simulink model "s5_Inverter_PSMG"  (R2019b)
settings: Solver=VariableStepAuto  StartTime=0.0  StopTime=10.0  RelTol=1e-3
libraries: powerlib x41, powerlib_meascontrol x7, simulink_extras x1
settings Model: Creator=MAHMUD  LastModifiedBy=MAHMUD

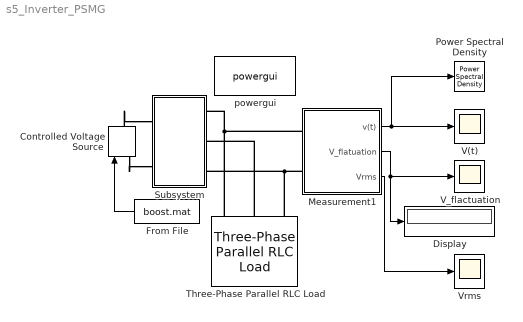
== system s5_Inverter_PSMG ==
  Controlled Voltage Source : powerlib/Electrical Sources/Controlled Voltage Source  Initialize=on  Source_Type=DC  Amplitude=0  Phase=0  Frequency=0  Measurements=None
      settings: SourceProductName=Simscape Electrical
  Display : Display
  From File : FromFile  FileName=boost.mat
  Measurement1 : Subsystem
  Power Spectral Density : simulink_extras/Additional Sinks/Power Spectral Density  npts=5000  fftpts=512  HowOften=500  sampleT=0.001
      settings: SourceProductName=Simulink  SourceProductBaseCode=SL
  Subsystem : Subsystem
  Three-Phase Parallel RLC Load : powerlib/Elements/Three-Phase Parallel RLC Load  LConnTagsString=A|B|C  Configuration=Y (grounded)  NominalVoltage=1000  Vabc=[1e3 1e3 1e3]  Vabcp=[1e3 1e3 1e3]  NominalFrequency=50  UnbalancedPower=off  ActivePower=16e3  InductivePower=100  CapacitivePower=100  Pabc=[10e3 9e3 11e3]  QLabc=[100 90 110]  QCabc=[100 90 110]  Pabcp=[10e3 9e3 11e3]  QLabcp=[100 90 110]  QCabcp=[100 90 110]  Measurements=None  LoadType=constant Z
      settings: SourceProductName=Simscape Electrical
  V(t) : Scope
  V_flactuation : Scope
  Vrms : Scope
  powergui : powerlib/powergui  Priority=1  SimulationMode=Continuous  SampleTime=50e-6  frequency=60  Iterations=50  frequencyindice=0  Pbase=100e6  ErrMax=1e-4  UnitsV=kV  UnitsW=MW  buscounter=0  FunctionMessages=off  echomessages=off  EnableUseOfTLC=off  CurrentSourceSwitches=off  DisableSnubberDevices=off  DisableRonSwitches=off  DisableVfSwitches=off  DisplayEquations=off  AutomaticDiscreteSolvers=off  SolverType=Tustin/Backward Euler (TBE)  Interpol=off  ExternalGateDelay=off  methode=off  Ts=100  x0status=blocks  SPID=on  SwTol=0  HookPort=off  NonlinearTolerance=1e-4  nMaxIteration=100  ContinueOnMaxIteration=off  RestoreLinks=warning  ResistiveCurrentMeasurement=off  Frange=[0:2:500]  Ylog=off  Xlog=on  ShowGrid=off  save=off  variable=ZData  structure=0  ZoomFFT=off  StartTime=0.0  cycles=1  DisplayStyle=1  fundamental=60  FreqAxis=off  MaxFrequency=1000  frequencyindicesteady=1  RmsSteady=1  display=off
      settings: SourceProductName=Simscape Electrical
  wires:
  From File/1 -> Controlled Voltage Source/1
  Measurement1/3(Vrms) -> Vrms/1
  Measurement1/2(V_flatuation) -> Display/1, V_flactuation/1
  Measurement1/1(v(t)) -> V(t)/1, Power Spectral Density/1
  connections:
  Controlled Voltage Source/RConn1 -- Subsystem/LConn1
  Controlled Voltage Source/LConn1 -- Subsystem/LConn2
  Three-Phase Parallel RLC Load/LConn1 -- Subsystem/RConn1 -- Measurement1/LConn1
  Three-Phase Parallel RLC Load/LConn2 -- Subsystem/RConn2
  Three-Phase Parallel RLC Load/LConn3 -- Subsystem/RConn3 -- Measurement1/LConn2

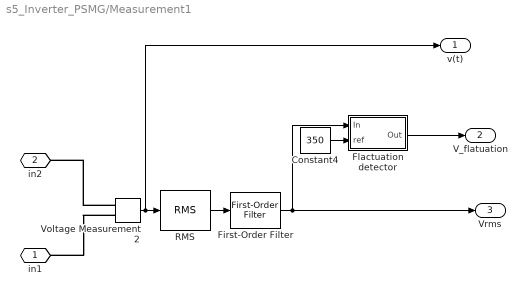
== system s5_Inverter_PSMG/Measurement1 ==
  Constant4 : Constant  Value=350
  First-Order Filter : powerlib_meascontrol/Filters/First-Order Filter  FilterType=Lowpass  Tc=100e-3  Ts=0  Initialize=off  Vac_Init=[0, 0, 50]  Vdc_Init=0  PlotResponse=off  FreqRange="[0,  200,  1]"
      settings: SourceProductName=Simscape Electrical
  Flactuation detector : Subsystem
  RMS : powerlib_meascontrol/Measurements/RMS  TrueRMS=on  Freq=50  RMSInit=210  Ts=0.001
      settings: SourceProductName=Simscape Electrical
  Voltage Measurement2 : powerlib/Measurements/Voltage Measurement  PhasorSimulation=off  OutputType=Complex  PSBequivalent=0
      settings: SourceProductName=Simscape Electrical
  in1 : PMIOPort  Side=Left
  in2 : PMIOPort  Port=2  Side=Left
  v(t) : Outport
  V_flatuation : Outport  Port=2
  Vrms : Outport  Port=3
  wires:
  Voltage Measurement2/1 -> v(t)/1, RMS/1
  First-Order Filter/1 -> Vrms/1, Flactuation detector/1(In)
  RMS/1 -> First-Order Filter/1
  Flactuation detector/1(Out) -> V_flatuation/1
  Constant4/1 -> Flactuation detector/2(ref)
  connections:
  Voltage Measurement2/LConn2 -- in1/RConn1
  Voltage Measurement2/LConn1 -- in2/RConn1

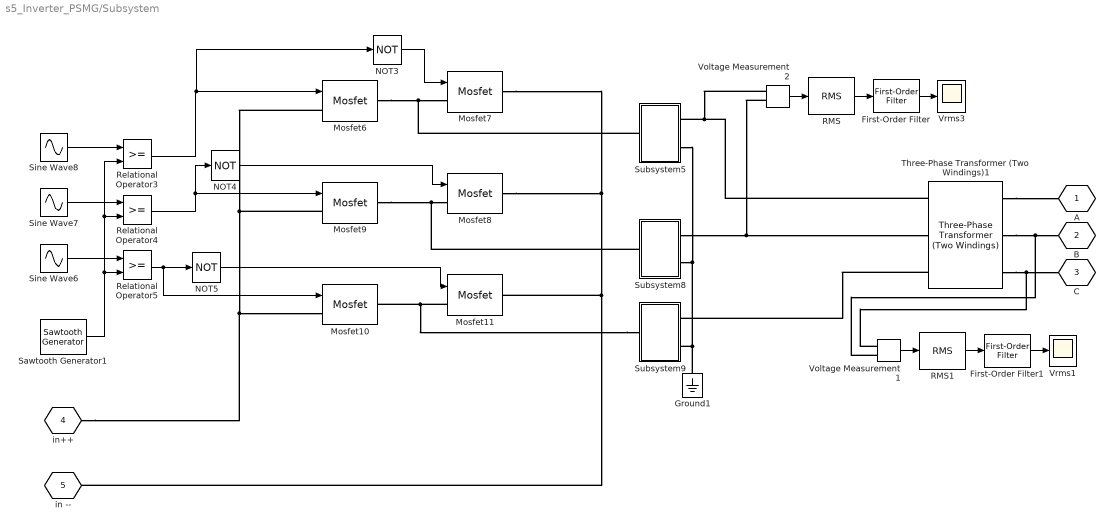
== system s5_Inverter_PSMG/Subsystem ==
  First-Order Filter : powerlib_meascontrol/Filters/First-Order Filter  FilterType=Lowpass  Tc=100e-3  Ts=0  Initialize=off  Vac_Init=[0, 0, 50]  Vdc_Init=0  PlotResponse=off  FreqRange="[0,  200,  1]"
      settings: SourceProductName=Simscape Electrical
  First-Order Filter1 : powerlib_meascontrol/Filters/First-Order Filter  FilterType=Lowpass  Tc=100e-3  Ts=0  Initialize=off  Vac_Init=[0, 0, 50]  Vdc_Init=0  PlotResponse=off  FreqRange="[0,  200,  1]"
      settings: SourceProductName=Simscape Electrical
  Ground1 : powerlib/Elements/Ground  LConnTagsString=a
      settings: SourceProductName=Simscape Electrical
  Mosfet{6..11} (6 alike) : powerlib/Power Electronics/Mosfet  Ron=0.1  Lon=0  Rd=0.01  Vfd=0  IC=0  Rs=1e5  Cs=inf  Measurements=off
      settings: SourceProductName=Simscape Electrical
  NOT3 : Logic  Operator=NOT  IconShape=distinctive  AllPortsSameDT=off  OutDataTypeStr=boolean
  NOT4 : Logic  Operator=NOT  IconShape=distinctive  AllPortsSameDT=off  OutDataTypeStr=boolean
  NOT5 : Logic  Operator=NOT  IconShape=distinctive  AllPortsSameDT=off  OutDataTypeStr=boolean
  RMS : powerlib_meascontrol/Measurements/RMS  TrueRMS=on  Freq=50  RMSInit=210  Ts=0.001
      settings: SourceProductName=Simscape Electrical
  RMS1 : powerlib_meascontrol/Measurements/RMS  TrueRMS=on  Freq=50  RMSInit=210  Ts=0.001
      settings: SourceProductName=Simscape Electrical
  Relational Operator3 : RelationalOperator  OutDataTypeStr=boolean  ZeroCross=off  RndMeth=Simplest
  Relational Operator4 : RelationalOperator  OutDataTypeStr=boolean  ZeroCross=off  RndMeth=Simplest
  Relational Operator5 : RelationalOperator  OutDataTypeStr=boolean  ZeroCross=off  RndMeth=Simplest
  Sawtooth Generator1 : powerlib_meascontrol/Pulse & Signal Generators/Sawtooth Generator  Freq=1e3  Phase=180  Ts=0
      settings: SourceProductName=Simscape Electrical
  Sine Wave6 : Sin  Frequency=2*pi*50  Phase=4*pi/3  SampleTime=0
  Sine Wave7 : Sin  Frequency=2*pi*50  Phase=2*pi/3  SampleTime=0
  Sine Wave8 : Sin  Frequency=2*pi*50  SampleTime=0
  Subsystem5 : Subsystem
  Subsystem8 : Subsystem
  Subsystem9 : Subsystem
  Three-Phase Transformer (Two Windings)1 : powerlib/Elements/Three-Phase Transformer (Two Windings)  Winding1Connection=Yg  Winding2Connection=Yg  CoreType=Three single-phase transformers  SetSaturation=off  Hysteresis=off  DataFile='hysteresis'  SetInitialFlux=off  Measurements=None  UNITS=pu  NominalPower=[ 16e3 , 50 ]  Winding1=[ 80 , 0.002 , 0.08 ]  Winding2=[ 400 , 0.002 , 0.08 ]  Rm=500  Lm=500  L0=0.5  Saturation=[ 0,0 ; 0.0024,1.2 ; 1.0,1.52 ]  InitialFluxes=[ 0.8 , -0.8 , 0.7 ]  BreakLoop=off  DiscreteSolver=Trapezoidal iterative  DataType=off  TransfoNumber=1
      settings: SourceProductName=Simscape Electrical
  Voltage Measurement1 : powerlib/Measurements/Voltage Measurement  PhasorSimulation=off  OutputType=Complex  PSBequivalent=0
      settings: SourceProductName=Simscape Electrical
  Voltage Measurement2 : powerlib/Measurements/Voltage Measurement  PhasorSimulation=off  OutputType=Complex  PSBequivalent=0
      settings: SourceProductName=Simscape Electrical
  Vrms1 : Scope
  Vrms3 : Scope
  A : PMIOPort  Tag=PMCPort  Side=Right
  B : PMIOPort  Tag=PMCPort  Port=2  Side=Right
  C : PMIOPort  Tag=PMCPort  Port=3  Side=Right
  in++ : PMIOPort  Tag=PMCPort  Port=4  Side=Left
  in -- : PMIOPort  Tag=PMCPort  Port=5  Side=Left
  wires:
  Relational Operator3/1 -> NOT3/1, Mosfet6/1
  Sine Wave7/1 -> Relational Operator4/1
  NOT4/1 -> Mosfet8/1
  Relational Operator5/1 -> Mosfet10/1, NOT5/1
  Relational Operator4/1 -> Mosfet9/1, NOT4/1
  Sine Wave8/1 -> Relational Operator3/1
  NOT5/1 -> Mosfet11/1
  NOT3/1 -> Mosfet7/1
  Sine Wave6/1 -> Relational Operator5/1
  Sawtooth Generator1/1 -> Relational Operator3/2, Relational Operator4/2, Relational Operator5/2
  Voltage Measurement2/1 -> RMS/1
  RMS/1 -> First-Order Filter/1
  First-Order Filter/1 -> Vrms3/1
  First-Order Filter1/1 -> Vrms1/1
  RMS1/1 -> First-Order Filter1/1
  Voltage Measurement1/1 -> RMS1/1
  connections:
  Subsystem5/RConn2 -- Ground1/LConn1 -- Subsystem9/RConn2 -- Subsystem8/RConn2
  Three-Phase Transformer (Two Windings)1/LConn3 -- Subsystem9/RConn1
  Subsystem8/LConn1 -- Mosfet9/RConn1 -- Mosfet8/LConn1
  Subsystem5/LConn1 -- Mosfet6/RConn1 -- Mosfet7/LConn1
  Mosfet6/LConn1 -- in++/RConn1 -- Mosfet10/LConn1 -- Mosfet9/LConn1
  Subsystem9/LConn1 -- Mosfet11/LConn1 -- Mosfet10/RConn1
  Mosfet11/RConn1 -- in --/RConn1 -- Mosfet7/RConn1 -- Mosfet8/RConn1
  Three-Phase Transformer (Two Windings)1/RConn2 -- Voltage Measurement1/LConn2 -- B/RConn1
  Three-Phase Transformer (Two Windings)1/LConn1 -- Voltage Measurement2/LConn1 -- Subsystem5/RConn1
  Subsystem8/RConn1 -- Voltage Measurement2/LConn2 -- Three-Phase Transformer (Two Windings)1/LConn2
  Three-Phase Transformer (Two Windings)1/RConn3 -- Voltage Measurement1/LConn1 -- C/RConn1
  Three-Phase Transformer (Two Windings)1/RConn1 -- A/RConn1

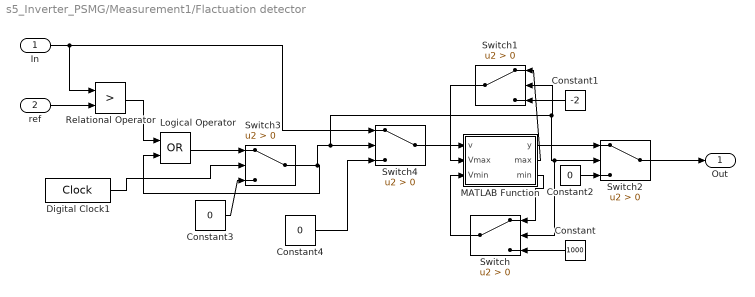
== system s5_Inverter_PSMG/Measurement1/Flactuation detector ==
  In : Inport
  ref : Inport  Port=2
  Constant : Constant  Value=1000
  Constant1 : Constant  Value=-2
  Constant2 : Constant  Value=0
  Constant3 : Constant  Value=0
  Constant4 : Constant  Value=0
  Digital Clock1 : DigitalClock
  Logical Operator : Logic  Operator=OR  AllPortsSameDT=off  OutDataTypeStr=boolean
  MATLAB Function : MATLAB Function  TreatAsAtomicUnit=on
  Relational Operator : RelationalOperator  Operator=>  OutDataTypeStr=boolean  ZeroCross=off  RndMeth=Simplest
  Switch{,1..4} (5 alike) : Switch  Criteria=u2 > Threshold  ZeroCross=off
  Out : Outport
  wires:
  Constant/1 -> Switch/3
  Switch1/1 -> MATLAB Function/2(Vmax)
  Constant1/1 -> Switch1/3
  MATLAB Function/1(y) -> Switch2/1
  MATLAB Function/3(min) -> Switch/1
  Switch2/1 -> Out/1
  MATLAB Function/2(max) -> Switch1/1
  Switch/1 -> MATLAB Function/3(Vmin)
  Constant2/1 -> Switch2/3
  Logical Operator/1 -> Switch3/1
  Switch3/1 -> Switch/2, Switch2/2, Switch1/2, Switch4/2, Logical Operator/2
  Constant3/1 -> Switch3/3
  Relational Operator/1 -> Logical Operator/1
  Switch4/1 -> MATLAB Function/1(v)
  In/1 -> Relational Operator/1, Switch4/1
  Digital Clock1/1 -> Switch3/2
  ref/1 -> Relational Operator/2
  Constant4/1 -> Switch4/3

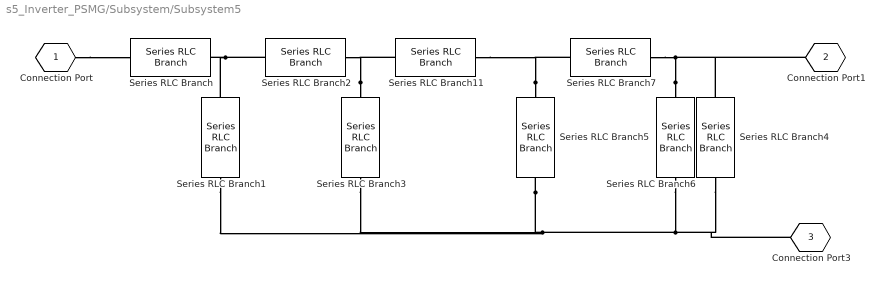
== system s5_Inverter_PSMG/Subsystem/Subsystem5 ==
  Series RLC Branch{,2,5..6} (4 alike) : powerlib/Elements/Series RLC Branch  LConnTagsString=__new0  RConnTagsString=__new0  BranchType=L  Resistance=1  Inductance=92e-3  SetiL0=off  InitialCurrent=0  Capacitance=1e-6  Setx0=off  InitialVoltage=0  Measurements=None
      settings: SourceProductName=Simscape Electrical
  Series RLC Branch1 : powerlib/Elements/Series RLC Branch  LConnTagsString=__new0  RConnTagsString=__new0  BranchType=C  Resistance=1  Inductance=1e-3  SetiL0=off  InitialCurrent=0  Capacitance=110e-6  Setx0=off  InitialVoltage=0  Measurements=None
      settings: SourceProductName=Simscape Electrical
  Series RLC Branch11 : powerlib/Elements/Series RLC Branch  LConnTagsString=__new0  RConnTagsString=__new0  BranchType=R  Resistance=1  Inductance=1e-3  SetiL0=off  InitialCurrent=0  Capacitance=110e-6  Setx0=off  InitialVoltage=0  Measurements=None
      settings: SourceProductName=Simscape Electrical
  Series RLC Branch3 : powerlib/Elements/Series RLC Branch  LConnTagsString=__new0  RConnTagsString=__new0  BranchType=R  Resistance=500  Inductance=1e-3  SetiL0=off  InitialCurrent=0  Capacitance=110e-6  Setx0=off  InitialVoltage=0  Measurements=None
      settings: SourceProductName=Simscape Electrical
  Series RLC Branch4 : powerlib/Elements/Series RLC Branch  LConnTagsString=__new0  RConnTagsString=__new0  BranchType=R  Resistance=10  Inductance=1e-3  SetiL0=off  InitialCurrent=0  Capacitance=110e-6  Setx0=off  InitialVoltage=0  Measurements=None
      settings: SourceProductName=Simscape Electrical
  Series RLC Branch7 : powerlib/Elements/Series RLC Branch  LConnTagsString=__new0  RConnTagsString=__new0  BranchType=C  Resistance=1  Inductance=1e-3  SetiL0=off  InitialCurrent=0  Capacitance=110e-6  Setx0=off  InitialVoltage=0  Measurements=None
      settings: SourceProductName=Simscape Electrical
  Connection Port : PMIOPort  Tag=PMCPort  Side=Left
  Connection Port1 : PMIOPort  Tag=PMCPort  Port=2  Side=Right
  Connection Port3 : PMIOPort  Tag=PMCPort  Port=3  Side=Right
  connections:
  Connection Port/RConn1 -- Series RLC Branch/LConn1
  Series RLC Branch/RConn1 -- Series RLC Branch2/LConn1 -- Series RLC Branch1/RConn1
  Series RLC Branch5/LConn1 -- Series RLC Branch11/RConn1 -- Series RLC Branch7/LConn1
  Series RLC Branch5/RConn1 -- Series RLC Branch6/RConn1 -- Series RLC Branch4/LConn1 -- Connection Port3/RConn1 -- Series RLC Branch3/LConn1 -- Series RLC Branch1/LConn1
  Series RLC Branch3/RConn1 -- Series RLC Branch11/LConn1 -- Series RLC Branch2/RConn1
  Series RLC Branch6/LConn1 -- Series RLC Branch4/RConn1 -- Connection Port1/RConn1 -- Series RLC Branch7/RConn1

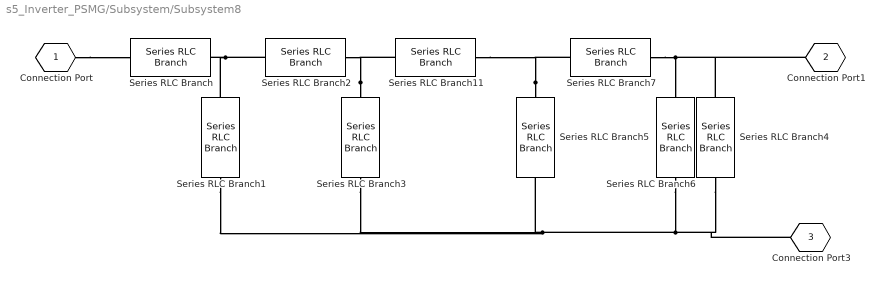
== system s5_Inverter_PSMG/Subsystem/Subsystem8 ==
  Series RLC Branch{,2,5..6} (4 alike) : powerlib/Elements/Series RLC Branch  LConnTagsString=__new0  RConnTagsString=__new0  BranchType=L  Resistance=1  Inductance=92e-3  SetiL0=off  InitialCurrent=0  Capacitance=1e-6  Setx0=off  InitialVoltage=0  Measurements=None
      settings: SourceProductName=Simscape Electrical
  Series RLC Branch1 : powerlib/Elements/Series RLC Branch  LConnTagsString=__new0  RConnTagsString=__new0  BranchType=C  Resistance=1  Inductance=1e-3  SetiL0=off  InitialCurrent=0  Capacitance=110e-6  Setx0=off  InitialVoltage=0  Measurements=None
      settings: SourceProductName=Simscape Electrical
  Series RLC Branch11 : powerlib/Elements/Series RLC Branch  LConnTagsString=__new0  RConnTagsString=__new0  BranchType=R  Resistance=1  Inductance=1e-3  SetiL0=off  InitialCurrent=0  Capacitance=110e-6  Setx0=off  InitialVoltage=0  Measurements=None
      settings: SourceProductName=Simscape Electrical
  Series RLC Branch3 : powerlib/Elements/Series RLC Branch  LConnTagsString=__new0  RConnTagsString=__new0  BranchType=R  Resistance=500  Inductance=1e-3  SetiL0=off  InitialCurrent=0  Capacitance=110e-6  Setx0=off  InitialVoltage=0  Measurements=None
      settings: SourceProductName=Simscape Electrical
  Series RLC Branch4 : powerlib/Elements/Series RLC Branch  LConnTagsString=__new0  RConnTagsString=__new0  BranchType=R  Resistance=10  Inductance=1e-3  SetiL0=off  InitialCurrent=0  Capacitance=110e-6  Setx0=off  InitialVoltage=0  Measurements=None
      settings: SourceProductName=Simscape Electrical
  Series RLC Branch7 : powerlib/Elements/Series RLC Branch  LConnTagsString=__new0  RConnTagsString=__new0  BranchType=C  Resistance=1  Inductance=1e-3  SetiL0=off  InitialCurrent=0  Capacitance=110e-6  Setx0=off  InitialVoltage=0  Measurements=None
      settings: SourceProductName=Simscape Electrical
  Connection Port : PMIOPort  Tag=PMCPort  Side=Left
  Connection Port1 : PMIOPort  Tag=PMCPort  Port=2  Side=Right
  Connection Port3 : PMIOPort  Tag=PMCPort  Port=3  Side=Right
  connections:
  Series RLC Branch7/RConn1 -- Series RLC Branch6/LConn1 -- Series RLC Branch4/RConn1 -- Connection Port1/RConn1
  Series RLC Branch3/RConn1 -- Series RLC Branch2/RConn1 -- Series RLC Branch11/LConn1
  Series RLC Branch6/RConn1 -- Series RLC Branch3/LConn1 -- Series RLC Branch1/LConn1 -- Series RLC Branch5/RConn1 -- Series RLC Branch4/LConn1 -- Connection Port3/RConn1
  Series RLC Branch5/LConn1 -- Series RLC Branch7/LConn1 -- Series RLC Branch11/RConn1
  Series RLC Branch1/RConn1 -- Series RLC Branch2/LConn1 -- Series RLC Branch/RConn1
  Connection Port/RConn1 -- Series RLC Branch/LConn1

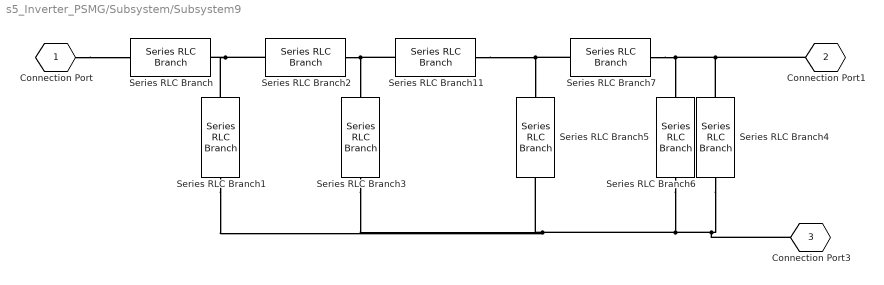
== system s5_Inverter_PSMG/Subsystem/Subsystem9 ==
  Series RLC Branch{,2,5..6} (4 alike) : powerlib/Elements/Series RLC Branch  LConnTagsString=__new0  RConnTagsString=__new0  BranchType=L  Resistance=1  Inductance=92e-3  SetiL0=off  InitialCurrent=0  Capacitance=1e-6  Setx0=off  InitialVoltage=0  Measurements=None
      settings: SourceProductName=Simscape Electrical
  Series RLC Branch1 : powerlib/Elements/Series RLC Branch  LConnTagsString=__new0  RConnTagsString=__new0  BranchType=C  Resistance=1  Inductance=1e-3  SetiL0=off  InitialCurrent=0  Capacitance=110e-6  Setx0=off  InitialVoltage=0  Measurements=None
      settings: SourceProductName=Simscape Electrical
  Series RLC Branch11 : powerlib/Elements/Series RLC Branch  LConnTagsString=__new0  RConnTagsString=__new0  BranchType=R  Resistance=1  Inductance=1e-3  SetiL0=off  InitialCurrent=0  Capacitance=110e-6  Setx0=off  InitialVoltage=0  Measurements=None
      settings: SourceProductName=Simscape Electrical
  Series RLC Branch3 : powerlib/Elements/Series RLC Branch  LConnTagsString=__new0  RConnTagsString=__new0  BranchType=R  Resistance=500  Inductance=1e-3  SetiL0=off  InitialCurrent=0  Capacitance=110e-6  Setx0=off  InitialVoltage=0  Measurements=None
      settings: SourceProductName=Simscape Electrical
  Series RLC Branch4 : powerlib/Elements/Series RLC Branch  LConnTagsString=__new0  RConnTagsString=__new0  BranchType=R  Resistance=10  Inductance=1e-3  SetiL0=off  InitialCurrent=0  Capacitance=110e-6  Setx0=off  InitialVoltage=0  Measurements=None
      settings: SourceProductName=Simscape Electrical
  Series RLC Branch7 : powerlib/Elements/Series RLC Branch  LConnTagsString=__new0  RConnTagsString=__new0  BranchType=C  Resistance=1  Inductance=1e-3  SetiL0=off  InitialCurrent=0  Capacitance=110e-6  Setx0=off  InitialVoltage=0  Measurements=None
      settings: SourceProductName=Simscape Electrical
  Connection Port : PMIOPort  Tag=PMCPort  Side=Left
  Connection Port1 : PMIOPort  Tag=PMCPort  Port=2  Side=Right
  Connection Port3 : PMIOPort  Tag=PMCPort  Port=3  Side=Right
  connections:
  Connection Port/RConn1 -- Series RLC Branch/LConn1
  Series RLC Branch/RConn1 -- Series RLC Branch2/LConn1 -- Series RLC Branch1/RConn1
  Series RLC Branch11/RConn1 -- Series RLC Branch7/LConn1 -- Series RLC Branch5/LConn1
  Connection Port3/RConn1 -- Series RLC Branch4/LConn1 -- Series RLC Branch5/RConn1 -- Series RLC Branch3/LConn1 -- Series RLC Branch1/LConn1 -- Series RLC Branch6/RConn1
  Series RLC Branch11/LConn1 -- Series RLC Branch2/RConn1 -- Series RLC Branch3/RConn1
  Connection Port1/RConn1 -- Series RLC Branch4/RConn1 -- Series RLC Branch6/LConn1 -- Series RLC Branch7/RConn1

== matlab function s5_Inverter_PSMG/Measurement1/Flactuation detector/MATLAB Function ==
  data: v input; y output; Vmax input; Vmin input; max output; min output
function [y,max,min] = fcn(v,Vmax,Vmin)
if(v>0)
    if(v<Vmin)
        min=v;
    else
        min=Vmin;
    end
    if(v>Vmax)
        max=v;
    else 
        max=Vmax;
    end
    y=Vmax-Vmin;
else
    min=0;
    max=0;
    y=0;
end
